simulink model "filpers"  (R2021a)
settings: Solver=VariableStepAuto  StartTime=0.0  StopTime=0.05  RelTol=1e-3
values from neighbouring files (symbols this model uses):
  C = 0.01    [examplebode.m]
  L = 0.01    [examplebode.m]
  R = 1    [examplebode.m]
settings Model: Creator=spbro  LastModifiedBy=spbro

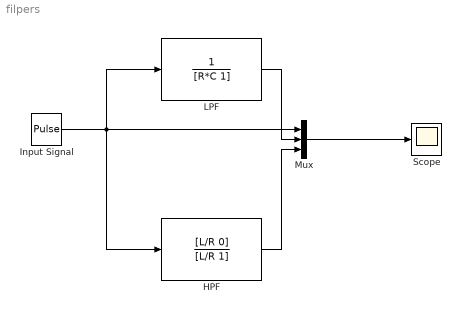
== system filpers ==
  HPF : TransferFcn  Numerator=[L/R 0]  Denominator=[L/R 1]
  Input Signal : DiscretePulseGenerator  PulseType=Time based  Period=0.005  PulseWidth=50
  LPF : TransferFcn  Denominator=[R*C 1]
  Mux : Mux  Inputs=3
  Scope : Scope
  wires:
  Input Signal/1 -> LPF/1, Mux/1, HPF/1
  LPF/1 -> Mux/2
  HPF/1 -> Mux/3
  Mux/1 -> Scope/1
